simulink library "ox_lib"  (Simulink 7.5)
settings: Solver=ode45  SolverMode=SingleTasking  StartTime=0.0  StopTime=10.0  RelTol=1e-3
PostLoadFcn:
  | % Stub definitions for mask variables
  | delay_depth=16;
  | n_bits=8;
  | bin_pt=7;
libraries: xbsIndex_r4 x493, casper_library x127, casper_library_misc x2, xps_library x2, casper_library_delays x1
(part 3 of 5)

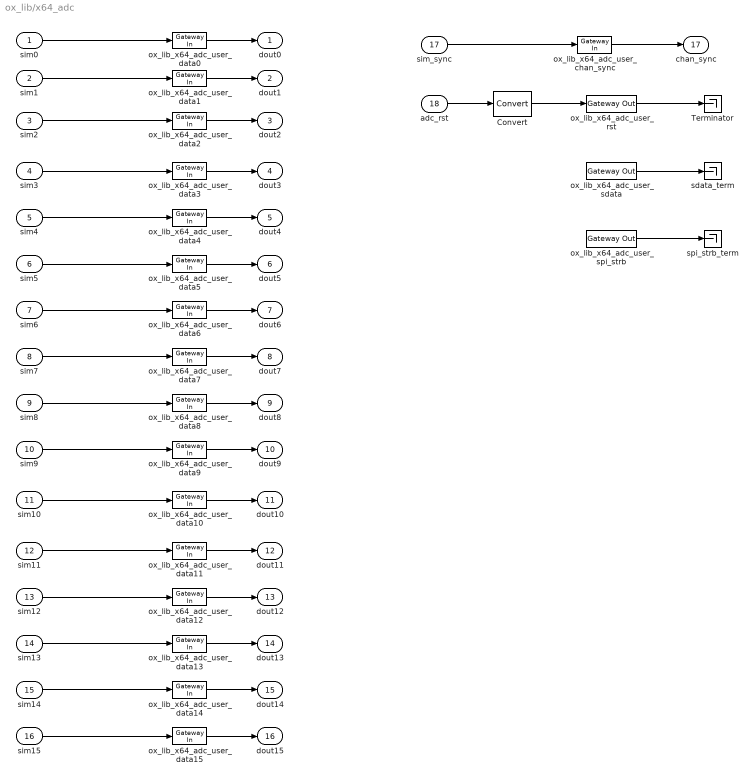
== system ox_lib/x64_adc ==
  sim0 : Inport
  sim1 : Inport  Port=2
  sim2 : Inport  Port=3
  sim3 : Inport  Port=4
  sim4 : Inport  Port=5
  sim5 : Inport  Port=6
  sim6 : Inport  Port=7
  sim7 : Inport  Port=8
  sim8 : Inport  Port=9
  sim9 : Inport  Port=10
  sim10 : Inport  Port=11
  sim11 : Inport  Port=12
  sim12 : Inport  Port=13
  sim13 : Inport  Port=14
  sim14 : Inport  Port=15
  sim15 : Inport  Port=16
  sim_sync : Inport  Port=17
  adc_rst : Inport  Port=18
  Convert : xbsIndex_r4/Convert  arith_type=Boolean  n_bits=16  bin_pt=14  quantization=Truncate  overflow=Wrap  latency=0  dbl_ovrd=off  pipeline=off  block_type=convert
      settings: block_version=11.4
  Terminator : Terminator
  ox_lib_x64_adc_user_chan_sync : xbsIndex_r4/Gateway In  arith_type=Unsigned  n_bits=8  bin_pt=0  quantization="Round  (unbiased: +/- Inf)"  overflow=Saturate  period=1  dbl_ovrd=off  timing_constraint=None  locs_specified=off  LOCs={}  hdl_port=on  block_type=gatewayin
      settings: infoedit="Gateway in block.  Converts inputs of type Simulink integer, double and fixed point to  Xilinx fixed point type.<br><br>Hardware notes:  In hardware these blocks become top level input ports."  block_version=11.4
  ox_lib_x64_adc_user_data{0..15} (16 alike) : xbsIndex_r4/Gateway In  arith_type="Signed  (2's comp)"  n_bits=12  bin_pt=11  quantization="Round  (unbiased: +/- Inf)"  overflow=Saturate  period=1  dbl_ovrd=off  timing_constraint=None  locs_specified=off  LOCs={}  hdl_port=on  block_type=gatewayin
      settings: infoedit="Gateway in block.  Converts inputs of type Simulink integer, double and fixed point to  Xilinx fixed point type.<br><br>Hardware notes:  In hardware these blocks become top level input ports."  block_version=11.4
  ox_lib_x64_adc_user_rst : xbsIndex_r4/Gateway Out  hdl_port=on  timing_constraint=None  locs_specified=off  LOCs={}  block_type=gatewayout
      settings: infoedit="Gateway out block.  Converts Xilinx fixed point inputs into ouputs of type Simulink integer, double, or fixed point.<br><br>Hardware notes:  In hardware these blocks become top level output ports or are discarded, depending on how they are configured."  block_version=11.4
  ox_lib_x64_adc_user_sdata : xbsIndex_r4/Gateway Out  hdl_port=on  timing_constraint=None  locs_specified=off  LOCs={}  block_type=gatewayout
      settings: infoedit="Gateway out block.  Converts Xilinx fixed point inputs into ouputs of type Simulink integer, double, or fixed point.<br><br>Hardware notes:  In hardware these blocks become top level output ports or are discarded, depending on how they are configured."  block_version=11.4
  ox_lib_x64_adc_user_spi_strb : xbsIndex_r4/Gateway Out  hdl_port=on  timing_constraint=None  locs_specified=off  LOCs={}  block_type=gatewayout
      settings: infoedit="Gateway out block.  Converts Xilinx fixed point inputs into ouputs of type Simulink integer, double, or fixed point.<br><br>Hardware notes:  In hardware these blocks become top level output ports or are discarded, depending on how they are configured."  block_version=11.4
  sdata_term : Terminator
  spi_strb_term : Terminator
  dout0 : Outport
  dout1 : Outport  Port=2
  dout2 : Outport  Port=3
  dout3 : Outport  Port=4
  dout4 : Outport  Port=5
  dout5 : Outport  Port=6
  dout6 : Outport  Port=7
  dout7 : Outport  Port=8
  dout8 : Outport  Port=9
  dout9 : Outport  Port=10
  dout10 : Outport  Port=11
  dout11 : Outport  Port=12
  dout12 : Outport  Port=13
  dout13 : Outport  Port=14
  dout14 : Outport  Port=15
  dout15 : Outport  Port=16
  chan_sync : Outport  Port=17
  wires:
  ox_lib_x64_adc_user_data1/1 -> dout1/1
  sim1/1 -> ox_lib_x64_adc_user_data1/1
  Convert/1 -> ox_lib_x64_adc_user_rst/1
  ox_lib_x64_adc_user_rst/1 -> Terminator/1
  adc_rst/1 -> Convert/1
  ox_lib_x64_adc_user_chan_sync/1 -> chan_sync/1
  sim_sync/1 -> ox_lib_x64_adc_user_chan_sync/1
  ox_lib_x64_adc_user_data15/1 -> dout15/1
  sim15/1 -> ox_lib_x64_adc_user_data15/1
  ox_lib_x64_adc_user_data14/1 -> dout14/1
  sim14/1 -> ox_lib_x64_adc_user_data14/1
  ox_lib_x64_adc_user_data13/1 -> dout13/1
  sim13/1 -> ox_lib_x64_adc_user_data13/1
  ox_lib_x64_adc_user_data12/1 -> dout12/1
  sim12/1 -> ox_lib_x64_adc_user_data12/1
  ox_lib_x64_adc_user_data11/1 -> dout11/1
  sim11/1 -> ox_lib_x64_adc_user_data11/1
  ox_lib_x64_adc_user_data10/1 -> dout10/1
  sim10/1 -> ox_lib_x64_adc_user_data10/1
  ox_lib_x64_adc_user_data9/1 -> dout9/1
  sim9/1 -> ox_lib_x64_adc_user_data9/1
  ox_lib_x64_adc_user_data8/1 -> dout8/1
  sim8/1 -> ox_lib_x64_adc_user_data8/1
  ox_lib_x64_adc_user_data7/1 -> dout7/1
  sim7/1 -> ox_lib_x64_adc_user_data7/1
  ox_lib_x64_adc_user_data6/1 -> dout6/1
  sim6/1 -> ox_lib_x64_adc_user_data6/1
  ox_lib_x64_adc_user_data5/1 -> dout5/1
  sim5/1 -> ox_lib_x64_adc_user_data5/1
  ox_lib_x64_adc_user_data4/1 -> dout4/1
  sim4/1 -> ox_lib_x64_adc_user_data4/1
  ox_lib_x64_adc_user_data3/1 -> dout3/1
  sim3/1 -> ox_lib_x64_adc_user_data3/1
  ox_lib_x64_adc_user_data2/1 -> dout2/1
  sim2/1 -> ox_lib_x64_adc_user_data2/1
  ox_lib_x64_adc_user_data0/1 -> dout0/1
  sim0/1 -> ox_lib_x64_adc_user_data0/1
  ? -> ox_lib_x64_adc_user_sdata/1
  ? -> ox_lib_x64_adc_user_spi_strb/1
  ox_lib_x64_adc_user_sdata/1 -> sdata_term/1
  ox_lib_x64_adc_user_spi_strb/1 -> spi_strb_term/1

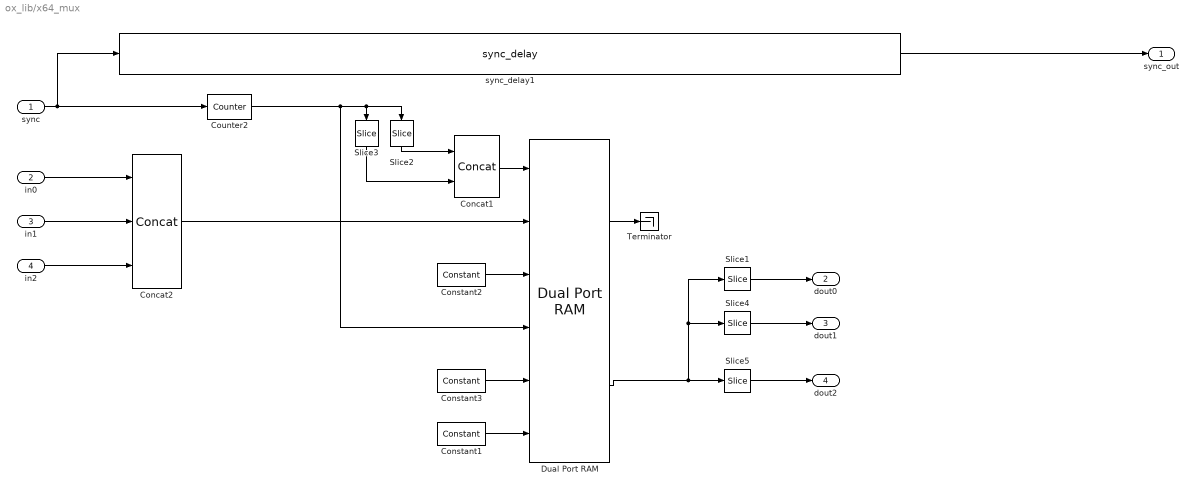
== system ox_lib/x64_mux ==
  sync : Inport  OutDataType=fixdt(1, 16)  OutScaling=2^0
  in0 : Inport  Port=2  OutDataType=fixdt(1, 16)  OutScaling=2^0
  in1 : Inport  Port=3  OutDataType=fixdt(1, 16)  OutScaling=2^0
  in2 : Inport  Port=4  OutDataType=fixdt(1, 16)  OutScaling=2^0
  Concat1 : xbsIndex_r4/Concat  num_inputs=2  dbl_ovrd=off  block_type=concat
  Concat2 : xbsIndex_r4/Concat  num_inputs=3  dbl_ovrd=off  block_type=concat
  Constant1 : xbsIndex_r4/Constant  arith_type=Boolean  const=0  n_bits=16  bin_pt=14  explicit_period=off  period=1  equ=P=C  opselect=C  inp2=PCIN>>17  opr=+  inp1=P  carry=CIN  dbl_ovrd=off  block_type=constant
      settings: block_version=11.4
  Constant2 : xbsIndex_r4/Constant  arith_type=Boolean  const=1  n_bits=16  bin_pt=14  explicit_period=on  period=1  equ=P=C  opselect=C  inp2=PCIN>>17  opr=+  inp1=P  carry=CIN  dbl_ovrd=off  block_type=constant
      settings: block_version=11.4
  Constant3 : xbsIndex_r4/Constant  arith_type=Unsigned  const=0  n_bits=36  bin_pt=0  explicit_period=on  period=1  equ=P=C  opselect=C  inp2=PCIN>>17  opr=+  inp1=P  carry=CIN  dbl_ovrd=off  block_type=constant
      settings: block_version=11.4
  Counter2 : xbsIndex_r4/Counter  cnt_type=Free Running  cnt_to=Inf  operation=Up  start_count=0  cnt_by_val=1  arith_type=Unsigned  n_bits=fft_len+2  bin_pt=0  load_pin=off  rst=on  en=off  explicit_period=on  period=1  dbl_ovrd=off  use_behavioral_HDL=off  implementation=Fabric  block_type=counter
      settings: block_version=11.4
  Dual Port RAM : xbsIndex_r4/Dual Port RAM  depth=2^(fft_len+2)  initVector=0  distributed_mem=Block RAM  init_a=0  init_b=0  rst_a=off  rst_b=off  en_a=off  en_b=off  latency=bram_lat  write_mode_A=Read Before Write  write_mode_B=Read Before Write  dbl_ovrd=off  optimize=Area  use_rpm=on  block_type=dpram
      settings: block_version=11.4
  Slice1 : xbsIndex_r4/Slice  nbits=12  boolean_output=off  mode=Lower Bit Location + Width  bit1=0  base1=MSB of Input  bit0=24  base0=LSB of Input  dbl_ovrd=off  block_type=slice
  Slice2 : xbsIndex_r4/Slice  nbits=2  boolean_output=off  mode=Lower Bit Location + Width  bit1=0  base1=MSB of Input  bit0=0  base0=LSB of Input  dbl_ovrd=off  block_type=slice
  Slice3 : xbsIndex_r4/Slice  nbits=fft_len  boolean_output=off  mode=Lower Bit Location + Width  bit1=0  base1=MSB of Input  bit0=2  base0=LSB of Input  dbl_ovrd=off  block_type=slice
  Slice4 : xbsIndex_r4/Slice  nbits=12  boolean_output=off  mode=Lower Bit Location + Width  bit1=0  base1=MSB of Input  bit0=12  base0=LSB of Input  dbl_ovrd=off  block_type=slice
  Slice5 : xbsIndex_r4/Slice  nbits=12  boolean_output=off  mode=Lower Bit Location + Width  bit1=0  base1=MSB of Input  bit0=0  base0=LSB of Input  dbl_ovrd=off  block_type=slice
  Terminator : Terminator
  sync_delay1 : casper_library/Delays/sync_delay  SystemSampleTime=-1  DelayLen=2^(fft_len+2)+bram_lat
  sync_out : Outport
  dout0 : Outport  Port=2
  dout1 : Outport  Port=3
  dout2 : Outport  Port=4
  wires:
  sync/1 -> Counter2/1, sync_delay1/1
  Counter2/1 -> Slice2/1, Slice3/1, Dual Port RAM/4
  Constant1/1 -> Dual Port RAM/6
  Constant3/1 -> Dual Port RAM/5
  sync_delay1/1 -> sync_out/1
  Dual Port RAM/1 -> Terminator/1
  in0/1 -> Concat2/1
  in1/1 -> Concat2/2
  in2/1 -> Concat2/3
  Slice2/1 -> Concat1/1
  Slice3/1 -> Concat1/2
  Concat1/1 -> Dual Port RAM/1
  Dual Port RAM/2 -> Slice5/1, Slice4/1, Slice1/1
  Slice5/1 -> dout2/1
  Slice1/1 -> dout0/1
  Slice4/1 -> dout1/1
  Concat2/1 -> Dual Port RAM/2
  Constant2/1 -> Dual Port RAM/3

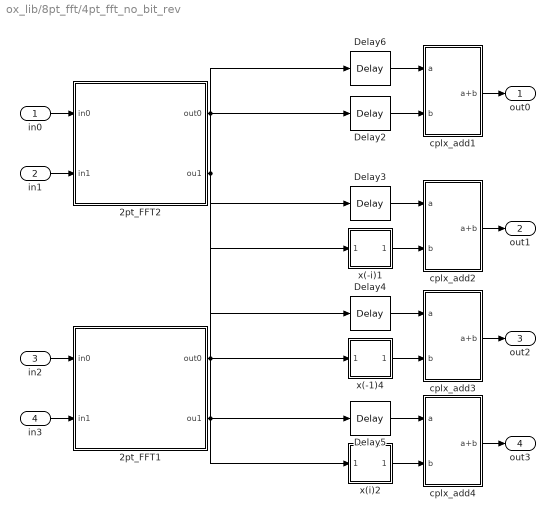
== system ox_lib/8pt_fft/4pt_fft_no_bit_rev ==
  in0 : Inport
  in1 : Inport  Port=2
  in2 : Inport  Port=3
  in3 : Inport  Port=4
  2pt_FFT1 : Subsystem
  2pt_FFT2 : Subsystem
  Delay{2..6} (5 alike) : xbsIndex_r4/Delay  en=off  latency=2  dbl_ovrd=off  reg_retiming=off  block_type=delay
      settings: block_version=11.4
  cplx_add1 : Subsystem  AncestorBlock=casper_library/Misc/complex_addsub  mask(cplx_add){BitWidth=8, add_latency=2}
      mask prompts: BitWidth "Bit Wdith"; add_latency "Add Latency"
  cplx_add2 : Subsystem  AncestorBlock=casper_library/Misc/complex_addsub  mask(cplx_add){BitWidth=8, add_latency=2}
      mask prompts: BitWidth "Bit Wdith"; add_latency "Add Latency"
  cplx_add3 : Subsystem  AncestorBlock=casper_library/Misc/complex_addsub  mask(cplx_add){BitWidth=8, add_latency=2}
      mask prompts: BitWidth "Bit Wdith"; add_latency "Add Latency"
  cplx_add4 : Subsystem  AncestorBlock=casper_library/Misc/complex_addsub  mask(cplx_add){BitWidth=8, add_latency=2}
      mask prompts: BitWidth "Bit Wdith"; add_latency "Add Latency"
  x(-1)4 : Subsystem
  x(-i)1 : Subsystem
  x(i)2 : Subsystem
  out0 : Outport
  out1 : Outport  Port=2
  out2 : Outport  Port=3
  out3 : Outport  Port=4
  wires:
  cplx_add4/1(a+b) -> out3/1
  in3/1 -> 2pt_FFT1/2(in1)
  in2/1 -> 2pt_FFT1/1(in0)
  cplx_add3/1(a+b) -> out2/1
  cplx_add2/1(a+b) -> out1/1
  in1/1 -> 2pt_FFT2/2(in1)
  in0/1 -> 2pt_FFT2/1(in0)
  cplx_add1/1(a+b) -> out0/1
  x(i)2/1(Out1) -> cplx_add4/2(b)
  Delay5/1 -> cplx_add4/1(a)
  x(-1)4/1(Out1) -> cplx_add3/2(b)
  Delay4/1 -> cplx_add3/1(a)
  x(-i)1/1(Out1) -> cplx_add2/2(b)
  Delay3/1 -> cplx_add2/1(a)
  Delay2/1 -> cplx_add1/2(b)
  Delay6/1 -> cplx_add1/1(a)
  2pt_FFT2/1(out0) -> Delay6/1, Delay4/1
  2pt_FFT2/2(ou1) -> Delay5/1, Delay3/1
  2pt_FFT1/1(out0) -> x(-1)4/1(In1), Delay2/1
  2pt_FFT1/2(ou1) -> x(-i)1/1(In1), x(i)2/1(In1)

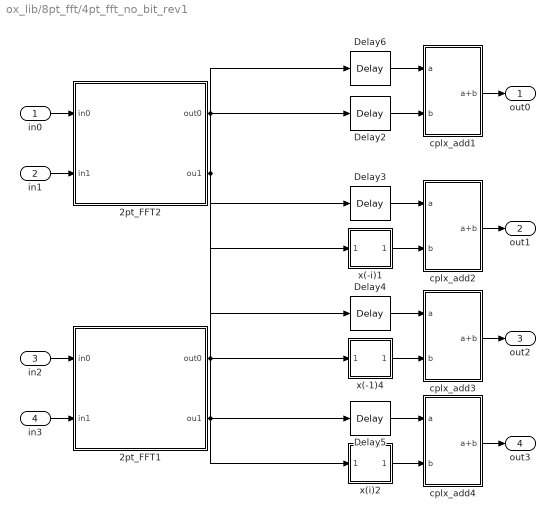
== system ox_lib/8pt_fft/4pt_fft_no_bit_rev1 ==
  in0 : Inport
  in1 : Inport  Port=2
  in2 : Inport  Port=3
  in3 : Inport  Port=4
  2pt_FFT1 : Subsystem
  2pt_FFT2 : Subsystem
  Delay{2..6} (5 alike) : xbsIndex_r4/Delay  en=off  latency=2  dbl_ovrd=off  reg_retiming=off  block_type=delay
      settings: block_version=11.4
  cplx_add1 : Subsystem  AncestorBlock=casper_library/Misc/complex_addsub  mask(cplx_add){BitWidth=8, add_latency=2}
      mask prompts: BitWidth "Bit Wdith"; add_latency "Add Latency"
  cplx_add2 : Subsystem  AncestorBlock=casper_library/Misc/complex_addsub  mask(cplx_add){BitWidth=8, add_latency=2}
      mask prompts: BitWidth "Bit Wdith"; add_latency "Add Latency"
  cplx_add3 : Subsystem  AncestorBlock=casper_library/Misc/complex_addsub  mask(cplx_add){BitWidth=8, add_latency=2}
      mask prompts: BitWidth "Bit Wdith"; add_latency "Add Latency"
  cplx_add4 : Subsystem  AncestorBlock=casper_library/Misc/complex_addsub  mask(cplx_add){BitWidth=8, add_latency=2}
      mask prompts: BitWidth "Bit Wdith"; add_latency "Add Latency"
  x(-1)4 : Subsystem
  x(-i)1 : Subsystem
  x(i)2 : Subsystem
  out0 : Outport
  out1 : Outport  Port=2
  out2 : Outport  Port=3
  out3 : Outport  Port=4
  wires:
  2pt_FFT1/2(ou1) -> x(i)2/1(In1), x(-i)1/1(In1)
  2pt_FFT1/1(out0) -> Delay2/1, x(-1)4/1(In1)
  2pt_FFT2/2(ou1) -> Delay3/1, Delay5/1
  2pt_FFT2/1(out0) -> Delay4/1, Delay6/1
  Delay6/1 -> cplx_add1/1(a)
  Delay2/1 -> cplx_add1/2(b)
  Delay3/1 -> cplx_add2/1(a)
  x(-i)1/1(Out1) -> cplx_add2/2(b)
  Delay4/1 -> cplx_add3/1(a)
  x(-1)4/1(Out1) -> cplx_add3/2(b)
  Delay5/1 -> cplx_add4/1(a)
  x(i)2/1(Out1) -> cplx_add4/2(b)
  cplx_add1/1(a+b) -> out0/1
  in0/1 -> 2pt_FFT2/1(in0)
  in1/1 -> 2pt_FFT2/2(in1)
  cplx_add2/1(a+b) -> out1/1
  cplx_add3/1(a+b) -> out2/1
  in2/1 -> 2pt_FFT1/1(in0)
  in3/1 -> 2pt_FFT1/2(in1)
  cplx_add4/1(a+b) -> out3/1

== system ox_lib/8pt_fft/cplx_add1 ==
  a : Inport  OutDataType=sfix(16)  OutScaling=2^0
  b : Inport  Port=2  OutDataType=sfix(16)  OutScaling=2^0
  AddSub : xbsIndex_r4/AddSub  mode=Addition  use_carryin=off  use_carryout=off  en=off  latency=add_latency  precision=Full  arith_type=Unsigned  n_bits=8  bin_pt=2  quantization=Truncate  overflow=Wrap  dbl_ovrd=off  use_behavioral_HDL=on  hw_selection=Fabric  pipelined=off  use_rpm=on  block_type=addsub
      settings: xl_area=[0, 0, 0, 0, 0, 0, 0]  block_version=9.1.01
  AddSub2 : xbsIndex_r4/AddSub  mode=Addition  use_carryin=off  use_carryout=off  en=off  latency=add_latency  precision=Full  arith_type=Unsigned  n_bits=8  bin_pt=2  quantization=Truncate  overflow=Wrap  dbl_ovrd=off  use_behavioral_HDL=on  hw_selection=Fabric  pipelined=off  use_rpm=on  block_type=addsub
      settings: xl_area=[0, 0, 0, 0, 0, 0, 0]  block_version=9.1.01
  Convert : xbsIndex_r4/Convert  arith_type="Signed  (2's comp)"  n_bits=BitWidth  bin_pt=BitWidth - 1  quantization="Round  (unbiased: +/- Inf)"  overflow=Saturate  latency=add_latency  dbl_ovrd=off  pipeline=off  block_type=convert
      settings: xl_area=[0, 0, 0, 0, 0, 0, 0]
  Convert2 : xbsIndex_r4/Convert  arith_type="Signed  (2's comp)"  n_bits=BitWidth  bin_pt=BitWidth - 1  quantization="Round  (unbiased: +/- Inf)"  overflow=Saturate  latency=add_latency  dbl_ovrd=off  pipeline=off  block_type=convert
      settings: xl_area=[0, 0, 0, 0, 0, 0, 0]
  Scale : xbsIndex_r4/Scale  scale_factor=-1  dbl_ovrd=off  block_type=scale
  Scale1 : xbsIndex_r4/Scale  scale_factor=-1  dbl_ovrd=off  block_type=scale
  c_to_ri : casper_library/Misc/c_to_ri  SystemSampleTime=-1  n_bits=BitWidth  bin_pt=BitWidth-1
      settings: AttributesFormatString=8_7 r/i
  c_to_ri1 : casper_library/Misc/c_to_ri  SystemSampleTime=-1  n_bits=BitWidth  bin_pt=BitWidth-1
      settings: AttributesFormatString=8_7 r/i
  ri_to_c : casper_library/Misc/ri_to_c  SystemSampleTime=-1
  a+b : Outport  OutDataType=sfix(16)  OutScaling=2^0
  wires:
  AddSub/1 -> Scale1/1
  AddSub2/1 -> Scale/1
  c_to_ri/1 -> AddSub/1
  c_to_ri/2 -> AddSub2/1
  c_to_ri1/1 -> AddSub/2
  c_to_ri1/2 -> AddSub2/2
  Convert/1 -> ri_to_c/1
  Convert2/1 -> ri_to_c/2
  a/1 -> c_to_ri/1
  ri_to_c/1 -> a+b/1
  b/1 -> c_to_ri1/1
  Scale1/1 -> Convert/1
  Scale/1 -> Convert2/1

== system ox_lib/8pt_fft/cplx_add2 ==
  a : Inport  OutDataType=sfix(16)  OutScaling=2^0
  b : Inport  Port=2  OutDataType=sfix(16)  OutScaling=2^0
  AddSub : xbsIndex_r4/AddSub  mode=Addition  use_carryin=off  use_carryout=off  en=off  latency=add_latency  precision=Full  arith_type=Unsigned  n_bits=8  bin_pt=2  quantization=Truncate  overflow=Wrap  dbl_ovrd=off  use_behavioral_HDL=on  hw_selection=Fabric  pipelined=off  use_rpm=on  block_type=addsub
      settings: xl_area=[0, 0, 0, 0, 0, 0, 0]  block_version=9.1.01
  AddSub2 : xbsIndex_r4/AddSub  mode=Addition  use_carryin=off  use_carryout=off  en=off  latency=add_latency  precision=Full  arith_type=Unsigned  n_bits=8  bin_pt=2  quantization=Truncate  overflow=Wrap  dbl_ovrd=off  use_behavioral_HDL=on  hw_selection=Fabric  pipelined=off  use_rpm=on  block_type=addsub
      settings: xl_area=[0, 0, 0, 0, 0, 0, 0]  block_version=9.1.01
  Convert : xbsIndex_r4/Convert  arith_type="Signed  (2's comp)"  n_bits=BitWidth  bin_pt=BitWidth - 1  quantization="Round  (unbiased: +/- Inf)"  overflow=Saturate  latency=add_latency  dbl_ovrd=off  pipeline=off  block_type=convert
      settings: xl_area=[0, 0, 0, 0, 0, 0, 0]
  Convert2 : xbsIndex_r4/Convert  arith_type="Signed  (2's comp)"  n_bits=BitWidth  bin_pt=BitWidth - 1  quantization="Round  (unbiased: +/- Inf)"  overflow=Saturate  latency=add_latency  dbl_ovrd=off  pipeline=off  block_type=convert
      settings: xl_area=[0, 0, 0, 0, 0, 0, 0]
  Scale : xbsIndex_r4/Scale  scale_factor=-1  dbl_ovrd=off  block_type=scale
  Scale1 : xbsIndex_r4/Scale  scale_factor=-1  dbl_ovrd=off  block_type=scale
  c_to_ri : casper_library/Misc/c_to_ri  SystemSampleTime=-1  n_bits=BitWidth  bin_pt=BitWidth-1
      settings: AttributesFormatString=8_7 r/i
  c_to_ri1 : casper_library/Misc/c_to_ri  SystemSampleTime=-1  n_bits=BitWidth  bin_pt=BitWidth-1
      settings: AttributesFormatString=8_7 r/i
  ri_to_c : casper_library/Misc/ri_to_c  SystemSampleTime=-1
  a+b : Outport  OutDataType=sfix(16)  OutScaling=2^0
  wires:
  Scale/1 -> Convert2/1
  Scale1/1 -> Convert/1
  b/1 -> c_to_ri1/1
  ri_to_c/1 -> a+b/1
  a/1 -> c_to_ri/1
  Convert2/1 -> ri_to_c/2
  Convert/1 -> ri_to_c/1
  c_to_ri1/2 -> AddSub2/2
  c_to_ri1/1 -> AddSub/2
  c_to_ri/2 -> AddSub2/1
  c_to_ri/1 -> AddSub/1
  AddSub2/1 -> Scale/1
  AddSub/1 -> Scale1/1

== system ox_lib/8pt_fft/cplx_add3 ==
  a : Inport  OutDataType=sfix(16)  OutScaling=2^0
  b : Inport  Port=2  OutDataType=sfix(16)  OutScaling=2^0
  AddSub : xbsIndex_r4/AddSub  mode=Addition  use_carryin=off  use_carryout=off  en=off  latency=add_latency  precision=Full  arith_type=Unsigned  n_bits=8  bin_pt=2  quantization=Truncate  overflow=Wrap  dbl_ovrd=off  use_behavioral_HDL=on  hw_selection=Fabric  pipelined=off  use_rpm=on  block_type=addsub
      settings: xl_area=[0, 0, 0, 0, 0, 0, 0]  block_version=9.1.01
  AddSub2 : xbsIndex_r4/AddSub  mode=Addition  use_carryin=off  use_carryout=off  en=off  latency=add_latency  precision=Full  arith_type=Unsigned  n_bits=8  bin_pt=2  quantization=Truncate  overflow=Wrap  dbl_ovrd=off  use_behavioral_HDL=on  hw_selection=Fabric  pipelined=off  use_rpm=on  block_type=addsub
      settings: xl_area=[0, 0, 0, 0, 0, 0, 0]  block_version=9.1.01
  Convert : xbsIndex_r4/Convert  arith_type="Signed  (2's comp)"  n_bits=BitWidth  bin_pt=BitWidth - 1  quantization="Round  (unbiased: +/- Inf)"  overflow=Saturate  latency=add_latency  dbl_ovrd=off  pipeline=off  block_type=convert
      settings: xl_area=[0, 0, 0, 0, 0, 0, 0]
  Convert2 : xbsIndex_r4/Convert  arith_type="Signed  (2's comp)"  n_bits=BitWidth  bin_pt=BitWidth - 1  quantization="Round  (unbiased: +/- Inf)"  overflow=Saturate  latency=add_latency  dbl_ovrd=off  pipeline=off  block_type=convert
      settings: xl_area=[0, 0, 0, 0, 0, 0, 0]
  Scale : xbsIndex_r4/Scale  scale_factor=-1  dbl_ovrd=off  block_type=scale
  Scale1 : xbsIndex_r4/Scale  scale_factor=-1  dbl_ovrd=off  block_type=scale
  c_to_ri : casper_library/Misc/c_to_ri  SystemSampleTime=-1  n_bits=BitWidth  bin_pt=BitWidth-1
      settings: AttributesFormatString=8_7 r/i
  c_to_ri1 : casper_library/Misc/c_to_ri  SystemSampleTime=-1  n_bits=BitWidth  bin_pt=BitWidth-1
      settings: AttributesFormatString=8_7 r/i
  ri_to_c : casper_library/Misc/ri_to_c  SystemSampleTime=-1
  a+b : Outport  OutDataType=sfix(16)  OutScaling=2^0
  wires:
  AddSub/1 -> Scale1/1
  AddSub2/1 -> Scale/1
  c_to_ri/1 -> AddSub/1
  c_to_ri/2 -> AddSub2/1
  c_to_ri1/1 -> AddSub/2
  c_to_ri1/2 -> AddSub2/2
  Convert/1 -> ri_to_c/1
  Convert2/1 -> ri_to_c/2
  a/1 -> c_to_ri/1
  ri_to_c/1 -> a+b/1
  b/1 -> c_to_ri1/1
  Scale1/1 -> Convert/1
  Scale/1 -> Convert2/1

== system ox_lib/8pt_fft/cplx_add4 ==
  a : Inport  OutDataType=sfix(16)  OutScaling=2^0
  b : Inport  Port=2  OutDataType=sfix(16)  OutScaling=2^0
  AddSub : xbsIndex_r4/AddSub  mode=Addition  use_carryin=off  use_carryout=off  en=off  latency=add_latency  precision=Full  arith_type=Unsigned  n_bits=8  bin_pt=2  quantization=Truncate  overflow=Wrap  dbl_ovrd=off  use_behavioral_HDL=on  hw_selection=Fabric  pipelined=off  use_rpm=on  block_type=addsub
      settings: xl_area=[0, 0, 0, 0, 0, 0, 0]  block_version=9.1.01
  AddSub2 : xbsIndex_r4/AddSub  mode=Addition  use_carryin=off  use_carryout=off  en=off  latency=add_latency  precision=Full  arith_type=Unsigned  n_bits=8  bin_pt=2  quantization=Truncate  overflow=Wrap  dbl_ovrd=off  use_behavioral_HDL=on  hw_selection=Fabric  pipelined=off  use_rpm=on  block_type=addsub
      settings: xl_area=[0, 0, 0, 0, 0, 0, 0]  block_version=9.1.01
  Convert : xbsIndex_r4/Convert  arith_type="Signed  (2's comp)"  n_bits=BitWidth  bin_pt=BitWidth - 1  quantization="Round  (unbiased: +/- Inf)"  overflow=Saturate  latency=add_latency  dbl_ovrd=off  pipeline=off  block_type=convert
      settings: xl_area=[0, 0, 0, 0, 0, 0, 0]
  Convert2 : xbsIndex_r4/Convert  arith_type="Signed  (2's comp)"  n_bits=BitWidth  bin_pt=BitWidth - 1  quantization="Round  (unbiased: +/- Inf)"  overflow=Saturate  latency=add_latency  dbl_ovrd=off  pipeline=off  block_type=convert
      settings: xl_area=[0, 0, 0, 0, 0, 0, 0]
  Scale : xbsIndex_r4/Scale  scale_factor=-1  dbl_ovrd=off  block_type=scale
  Scale1 : xbsIndex_r4/Scale  scale_factor=-1  dbl_ovrd=off  block_type=scale
  c_to_ri : casper_library/Misc/c_to_ri  SystemSampleTime=-1  n_bits=BitWidth  bin_pt=BitWidth-1
      settings: AttributesFormatString=8_7 r/i
  c_to_ri1 : casper_library/Misc/c_to_ri  SystemSampleTime=-1  n_bits=BitWidth  bin_pt=BitWidth-1
      settings: AttributesFormatString=8_7 r/i
  ri_to_c : casper_library/Misc/ri_to_c  SystemSampleTime=-1
  a+b : Outport  OutDataType=sfix(16)  OutScaling=2^0
  wires:
  Scale/1 -> Convert2/1
  Scale1/1 -> Convert/1
  b/1 -> c_to_ri1/1
  ri_to_c/1 -> a+b/1
  a/1 -> c_to_ri/1
  Convert2/1 -> ri_to_c/2
  Convert/1 -> ri_to_c/1
  c_to_ri1/2 -> AddSub2/2
  c_to_ri1/1 -> AddSub/2
  c_to_ri/2 -> AddSub2/1
  c_to_ri/1 -> AddSub/1
  AddSub2/1 -> Scale/1
  AddSub/1 -> Scale1/1

== system ox_lib/8pt_fft/cplx_add5 ==
  a : Inport  OutDataType=sfix(16)  OutScaling=2^0
  b : Inport  Port=2  OutDataType=sfix(16)  OutScaling=2^0
  AddSub : xbsIndex_r4/AddSub  mode=Addition  use_carryin=off  use_carryout=off  en=off  latency=add_latency  precision=Full  arith_type=Unsigned  n_bits=8  bin_pt=2  quantization=Truncate  overflow=Wrap  dbl_ovrd=off  use_behavioral_HDL=on  hw_selection=Fabric  pipelined=off  use_rpm=on  block_type=addsub
      settings: xl_area=[0, 0, 0, 0, 0, 0, 0]  block_version=9.1.01
  AddSub2 : xbsIndex_r4/AddSub  mode=Addition  use_carryin=off  use_carryout=off  en=off  latency=add_latency  precision=Full  arith_type=Unsigned  n_bits=8  bin_pt=2  quantization=Truncate  overflow=Wrap  dbl_ovrd=off  use_behavioral_HDL=on  hw_selection=Fabric  pipelined=off  use_rpm=on  block_type=addsub
      settings: xl_area=[0, 0, 0, 0, 0, 0, 0]  block_version=9.1.01
  Convert : xbsIndex_r4/Convert  arith_type="Signed  (2's comp)"  n_bits=BitWidth  bin_pt=BitWidth - 1  quantization="Round  (unbiased: +/- Inf)"  overflow=Saturate  latency=add_latency  dbl_ovrd=off  pipeline=off  block_type=convert
      settings: xl_area=[0, 0, 0, 0, 0, 0, 0]
  Convert2 : xbsIndex_r4/Convert  arith_type="Signed  (2's comp)"  n_bits=BitWidth  bin_pt=BitWidth - 1  quantization="Round  (unbiased: +/- Inf)"  overflow=Saturate  latency=add_latency  dbl_ovrd=off  pipeline=off  block_type=convert
      settings: xl_area=[0, 0, 0, 0, 0, 0, 0]
  Scale : xbsIndex_r4/Scale  scale_factor=-1  dbl_ovrd=off  block_type=scale
  Scale1 : xbsIndex_r4/Scale  scale_factor=-1  dbl_ovrd=off  block_type=scale
  c_to_ri : casper_library/Misc/c_to_ri  SystemSampleTime=-1  n_bits=BitWidth  bin_pt=BitWidth-1
      settings: AttributesFormatString=8_7 r/i
  c_to_ri1 : casper_library/Misc/c_to_ri  SystemSampleTime=-1  n_bits=BitWidth  bin_pt=BitWidth-1
      settings: AttributesFormatString=8_7 r/i
  ri_to_c : casper_library/Misc/ri_to_c  SystemSampleTime=-1
  a+b : Outport  OutDataType=sfix(16)  OutScaling=2^0
  wires:
  AddSub/1 -> Scale1/1
  AddSub2/1 -> Scale/1
  c_to_ri/1 -> AddSub/1
  c_to_ri/2 -> AddSub2/1
  c_to_ri1/1 -> AddSub/2
  c_to_ri1/2 -> AddSub2/2
  Convert/1 -> ri_to_c/1
  Convert2/1 -> ri_to_c/2
  a/1 -> c_to_ri/1
  ri_to_c/1 -> a+b/1
  b/1 -> c_to_ri1/1
  Scale1/1 -> Convert/1
  Scale/1 -> Convert2/1

== system ox_lib/8pt_fft/cplx_add6 ==
  a : Inport  OutDataType=sfix(16)  OutScaling=2^0
  b : Inport  Port=2  OutDataType=sfix(16)  OutScaling=2^0
  AddSub : xbsIndex_r4/AddSub  mode=Addition  use_carryin=off  use_carryout=off  en=off  latency=add_latency  precision=Full  arith_type=Unsigned  n_bits=8  bin_pt=2  quantization=Truncate  overflow=Wrap  dbl_ovrd=off  use_behavioral_HDL=on  hw_selection=Fabric  pipelined=off  use_rpm=on  block_type=addsub
      settings: xl_area=[0, 0, 0, 0, 0, 0, 0]  block_version=9.1.01
  AddSub2 : xbsIndex_r4/AddSub  mode=Addition  use_carryin=off  use_carryout=off  en=off  latency=add_latency  precision=Full  arith_type=Unsigned  n_bits=8  bin_pt=2  quantization=Truncate  overflow=Wrap  dbl_ovrd=off  use_behavioral_HDL=on  hw_selection=Fabric  pipelined=off  use_rpm=on  block_type=addsub
      settings: xl_area=[0, 0, 0, 0, 0, 0, 0]  block_version=9.1.01
  Convert : xbsIndex_r4/Convert  arith_type="Signed  (2's comp)"  n_bits=BitWidth  bin_pt=BitWidth - 1  quantization="Round  (unbiased: +/- Inf)"  overflow=Saturate  latency=add_latency  dbl_ovrd=off  pipeline=off  block_type=convert
      settings: xl_area=[0, 0, 0, 0, 0, 0, 0]
  Convert2 : xbsIndex_r4/Convert  arith_type="Signed  (2's comp)"  n_bits=BitWidth  bin_pt=BitWidth - 1  quantization="Round  (unbiased: +/- Inf)"  overflow=Saturate  latency=add_latency  dbl_ovrd=off  pipeline=off  block_type=convert
      settings: xl_area=[0, 0, 0, 0, 0, 0, 0]
  Scale : xbsIndex_r4/Scale  scale_factor=-1  dbl_ovrd=off  block_type=scale
  Scale1 : xbsIndex_r4/Scale  scale_factor=-1  dbl_ovrd=off  block_type=scale
  c_to_ri : casper_library/Misc/c_to_ri  SystemSampleTime=-1  n_bits=BitWidth  bin_pt=BitWidth-1
      settings: AttributesFormatString=8_7 r/i
  c_to_ri1 : casper_library/Misc/c_to_ri  SystemSampleTime=-1  n_bits=BitWidth  bin_pt=BitWidth-1
      settings: AttributesFormatString=8_7 r/i
  ri_to_c : casper_library/Misc/ri_to_c  SystemSampleTime=-1
  a+b : Outport  OutDataType=sfix(16)  OutScaling=2^0
  wires:
  Scale/1 -> Convert2/1
  Scale1/1 -> Convert/1
  b/1 -> c_to_ri1/1
  ri_to_c/1 -> a+b/1
  a/1 -> c_to_ri/1
  Convert2/1 -> ri_to_c/2
  Convert/1 -> ri_to_c/1
  c_to_ri1/2 -> AddSub2/2
  c_to_ri1/1 -> AddSub/2
  c_to_ri/2 -> AddSub2/1
  c_to_ri/1 -> AddSub/1
  AddSub2/1 -> Scale/1
  AddSub/1 -> Scale1/1

== system ox_lib/8pt_fft/cplx_add7 ==
  a : Inport  OutDataType=sfix(16)  OutScaling=2^0
  b : Inport  Port=2  OutDataType=sfix(16)  OutScaling=2^0
  AddSub : xbsIndex_r4/AddSub  mode=Addition  use_carryin=off  use_carryout=off  en=off  latency=add_latency  precision=Full  arith_type=Unsigned  n_bits=8  bin_pt=2  quantization=Truncate  overflow=Wrap  dbl_ovrd=off  use_behavioral_HDL=on  hw_selection=Fabric  pipelined=off  use_rpm=on  block_type=addsub
      settings: xl_area=[0, 0, 0, 0, 0, 0, 0]  block_version=9.1.01
  AddSub2 : xbsIndex_r4/AddSub  mode=Addition  use_carryin=off  use_carryout=off  en=off  latency=add_latency  precision=Full  arith_type=Unsigned  n_bits=8  bin_pt=2  quantization=Truncate  overflow=Wrap  dbl_ovrd=off  use_behavioral_HDL=on  hw_selection=Fabric  pipelined=off  use_rpm=on  block_type=addsub
      settings: xl_area=[0, 0, 0, 0, 0, 0, 0]  block_version=9.1.01
  Convert : xbsIndex_r4/Convert  arith_type="Signed  (2's comp)"  n_bits=BitWidth  bin_pt=BitWidth - 1  quantization="Round  (unbiased: +/- Inf)"  overflow=Saturate  latency=add_latency  dbl_ovrd=off  pipeline=off  block_type=convert
      settings: xl_area=[0, 0, 0, 0, 0, 0, 0]
  Convert2 : xbsIndex_r4/Convert  arith_type="Signed  (2's comp)"  n_bits=BitWidth  bin_pt=BitWidth - 1  quantization="Round  (unbiased: +/- Inf)"  overflow=Saturate  latency=add_latency  dbl_ovrd=off  pipeline=off  block_type=convert
      settings: xl_area=[0, 0, 0, 0, 0, 0, 0]
  Scale : xbsIndex_r4/Scale  scale_factor=-1  dbl_ovrd=off  block_type=scale
  Scale1 : xbsIndex_r4/Scale  scale_factor=-1  dbl_ovrd=off  block_type=scale
  c_to_ri : casper_library/Misc/c_to_ri  SystemSampleTime=-1  n_bits=BitWidth  bin_pt=BitWidth-1
      settings: AttributesFormatString=8_7 r/i
  c_to_ri1 : casper_library/Misc/c_to_ri  SystemSampleTime=-1  n_bits=BitWidth  bin_pt=BitWidth-1
      settings: AttributesFormatString=8_7 r/i
  ri_to_c : casper_library/Misc/ri_to_c  SystemSampleTime=-1
  a+b : Outport  OutDataType=sfix(16)  OutScaling=2^0
  wires:
  AddSub/1 -> Scale1/1
  AddSub2/1 -> Scale/1
  c_to_ri/1 -> AddSub/1
  c_to_ri/2 -> AddSub2/1
  c_to_ri1/1 -> AddSub/2
  c_to_ri1/2 -> AddSub2/2
  Convert/1 -> ri_to_c/1
  Convert2/1 -> ri_to_c/2
  a/1 -> c_to_ri/1
  ri_to_c/1 -> a+b/1
  b/1 -> c_to_ri1/1
  Scale1/1 -> Convert/1
  Scale/1 -> Convert2/1

== system ox_lib/8pt_fft/cplx_add8 ==
  a : Inport  OutDataType=sfix(16)  OutScaling=2^0
  b : Inport  Port=2  OutDataType=sfix(16)  OutScaling=2^0
  AddSub : xbsIndex_r4/AddSub  mode=Addition  use_carryin=off  use_carryout=off  en=off  latency=add_latency  precision=Full  arith_type=Unsigned  n_bits=8  bin_pt=2  quantization=Truncate  overflow=Wrap  dbl_ovrd=off  use_behavioral_HDL=on  hw_selection=Fabric  pipelined=off  use_rpm=on  block_type=addsub
      settings: xl_area=[0, 0, 0, 0, 0, 0, 0]  block_version=9.1.01
  AddSub2 : xbsIndex_r4/AddSub  mode=Addition  use_carryin=off  use_carryout=off  en=off  latency=add_latency  precision=Full  arith_type=Unsigned  n_bits=8  bin_pt=2  quantization=Truncate  overflow=Wrap  dbl_ovrd=off  use_behavioral_HDL=on  hw_selection=Fabric  pipelined=off  use_rpm=on  block_type=addsub
      settings: xl_area=[0, 0, 0, 0, 0, 0, 0]  block_version=9.1.01
  Convert : xbsIndex_r4/Convert  arith_type="Signed  (2's comp)"  n_bits=BitWidth  bin_pt=BitWidth - 1  quantization="Round  (unbiased: +/- Inf)"  overflow=Saturate  latency=add_latency  dbl_ovrd=off  pipeline=off  block_type=convert
      settings: xl_area=[0, 0, 0, 0, 0, 0, 0]
  Convert2 : xbsIndex_r4/Convert  arith_type="Signed  (2's comp)"  n_bits=BitWidth  bin_pt=BitWidth - 1  quantization="Round  (unbiased: +/- Inf)"  overflow=Saturate  latency=add_latency  dbl_ovrd=off  pipeline=off  block_type=convert
      settings: xl_area=[0, 0, 0, 0, 0, 0, 0]
  Scale : xbsIndex_r4/Scale  scale_factor=-1  dbl_ovrd=off  block_type=scale
  Scale1 : xbsIndex_r4/Scale  scale_factor=-1  dbl_ovrd=off  block_type=scale
  c_to_ri : casper_library/Misc/c_to_ri  SystemSampleTime=-1  n_bits=BitWidth  bin_pt=BitWidth-1
      settings: AttributesFormatString=8_7 r/i
  c_to_ri1 : casper_library/Misc/c_to_ri  SystemSampleTime=-1  n_bits=BitWidth  bin_pt=BitWidth-1
      settings: AttributesFormatString=8_7 r/i
  ri_to_c : casper_library/Misc/ri_to_c  SystemSampleTime=-1
  a+b : Outport  OutDataType=sfix(16)  OutScaling=2^0
  wires:
  Scale/1 -> Convert2/1
  Scale1/1 -> Convert/1
  b/1 -> c_to_ri1/1
  ri_to_c/1 -> a+b/1
  a/1 -> c_to_ri/1
  Convert2/1 -> ri_to_c/2
  Convert/1 -> ri_to_c/1
  c_to_ri1/2 -> AddSub2/2
  c_to_ri1/1 -> AddSub/2
  c_to_ri/2 -> AddSub2/1
  c_to_ri/1 -> AddSub/1
  AddSub2/1 -> Scale/1
  AddSub/1 -> Scale1/1

== system ox_lib/8pt_fft/twid1 ==
  In1 : Inport  OutDataType=sfix(16)  OutScaling=2^0
  cmult : Subsystem  AncestorBlock=casper_library/Multipliers/cmult  mask(Complex Multiplier (4 real multipliers)){n_bits_a=8, bin_pt_a=7, n_bits_b=8, bin_pt_b=7, n_bits_ab=8, bin_pt_ab=7, quantization=Round  (unbiased: +/- Inf), overflow=Saturate, mult_latency=3, add_latency=2}
      mask prompts: n_bits_a "Number of Bits 'a'"; bin_pt_a "Binary Point 'a'"; n_bits_b "Number of Bits 'b'"; bin_pt_b "Binary Point 'b'"; n_bits_ab "Number of Bits 'ab'"; bin_pt_ab "Binary Point 'ab'"; mult_latency "Multiplier Latency"; add_latency "Adder Latency"
      mask help:
      | This block multiplies two complex numbers using 4 real multipliers and 2 real adders.
      |
      | Latency = multiplier latency + adder latency.
      mask init:
      | cmult_init(gcb, ...
      |     'n_bits_a',n_bits_a, ...
      |     'bin_pt_a',bin_pt_a, ...
      |     'n_bits_b',n_bits_b, ...
      |     'bin_pt_b',bin_pt_b, ...
      |     'n_bits_ab',n_bits_ab, ...
      |     'bin_pt_ab',bin_pt_ab, ...
      |     'quantization',quantization, ...
      |     'overflow', overflow,...
      |     'mult_latency', mult_latency, ...
      |     'add_latency', add_latency);
      settings: AttributesFormatString=|
      | 8_7 * 8_7 ==> 8_7
      | round inf, saturate
      |  Latency: 8
      mask StyleString: edit,edit,edit,edit,edit,edit,popup(Truncate|Round  (unbiased: +/- Inf)|Round  (unbiased: Even Values)),popup(Wrap|Saturate|Error),edit,edit
  im : xbsIndex_r4/Constant  arith_type=Signed (2's comp)  const=sin(phase)  n_bits=8  bin_pt=7  explicit_period=on  period=1  equ=P=C  opselect=C  inp2=PCIN>>17  opr=+  inp1=P  carry=CIN  dbl_ovrd=off  block_type=constant
      settings: block_version=11.4
  re : xbsIndex_r4/Constant  arith_type=Signed (2's comp)  const=cos(phase)  n_bits=8  bin_pt=7  explicit_period=on  period=1  equ=P=C  opselect=C  inp2=PCIN>>17  opr=+  inp1=P  carry=CIN  dbl_ovrd=off  block_type=constant
      settings: block_version=11.4
  ri_to_c1 : casper_library/Misc/ri_to_c  SystemSampleTime=-1
  Out1 : Outport  OutDataType=sfix(16)  OutScaling=2^0
  wires:
  cmult/1(ab) -> Out1/1
  In1/1 -> cmult/1(a)
  ri_to_c1/1 -> cmult/2(b)
  im/1 -> ri_to_c1/2
  re/1 -> ri_to_c1/1

== system ox_lib/8pt_fft/twid2 ==
  In1 : Inport  OutDataType=sfix(16)  OutScaling=2^0
  cmult : Subsystem  AncestorBlock=casper_library/Multipliers/cmult  mask(Complex Multiplier (4 real multipliers)){n_bits_a=8, bin_pt_a=7, n_bits_b=8, bin_pt_b=7, n_bits_ab=8, bin_pt_ab=7, quantization=Round  (unbiased: +/- Inf), overflow=Saturate, mult_latency=3, add_latency=2}
      mask prompts: n_bits_a "Number of Bits 'a'"; bin_pt_a "Binary Point 'a'"; n_bits_b "Number of Bits 'b'"; bin_pt_b "Binary Point 'b'"; n_bits_ab "Number of Bits 'ab'"; bin_pt_ab "Binary Point 'ab'"; mult_latency "Multiplier Latency"; add_latency "Adder Latency"
      mask help:
      | This block multiplies two complex numbers using 4 real multipliers and 2 real adders.
      |
      | Latency = multiplier latency + adder latency.
      mask init: same as ox_lib/8pt_fft/twid1/cmult
      settings: AttributesFormatString=|
      | 8_7 * 8_7 ==> 8_7
      | round inf, saturate
      |  Latency: 8
      mask StyleString: edit,edit,edit,edit,edit,edit,popup(Truncate|Round  (unbiased: +/- Inf)|Round  (unbiased: Even Values)),popup(Wrap|Saturate|Error),edit,edit
  im : xbsIndex_r4/Constant  arith_type=Signed (2's comp)  const=sin(phase)  n_bits=8  bin_pt=7  explicit_period=on  period=1  equ=P=C  opselect=C  inp2=PCIN>>17  opr=+  inp1=P  carry=CIN  dbl_ovrd=off  block_type=constant
      settings: block_version=11.4
  re : xbsIndex_r4/Constant  arith_type=Signed (2's comp)  const=cos(phase)  n_bits=8  bin_pt=7  explicit_period=on  period=1  equ=P=C  opselect=C  inp2=PCIN>>17  opr=+  inp1=P  carry=CIN  dbl_ovrd=off  block_type=constant
      settings: block_version=11.4
  ri_to_c1 : casper_library/Misc/ri_to_c  SystemSampleTime=-1
  Out1 : Outport  OutDataType=sfix(16)  OutScaling=2^0
  wires:
  re/1 -> ri_to_c1/1
  im/1 -> ri_to_c1/2
  ri_to_c1/1 -> cmult/2(b)
  In1/1 -> cmult/1(a)
  cmult/1(ab) -> Out1/1

== system ox_lib/8pt_fft/twid3 ==
  In1 : Inport  OutDataType=sfix(16)  OutScaling=2^0
  cmult : Subsystem  AncestorBlock=casper_library/Multipliers/cmult  mask(Complex Multiplier (4 real multipliers)){n_bits_a=8, bin_pt_a=7, n_bits_b=8, bin_pt_b=7, n_bits_ab=8, bin_pt_ab=7, quantization=Round  (unbiased: +/- Inf), overflow=Saturate, mult_latency=3, add_latency=2}
      mask prompts: n_bits_a "Number of Bits 'a'"; bin_pt_a "Binary Point 'a'"; n_bits_b "Number of Bits 'b'"; bin_pt_b "Binary Point 'b'"; n_bits_ab "Number of Bits 'ab'"; bin_pt_ab "Binary Point 'ab'"; mult_latency "Multiplier Latency"; add_latency "Adder Latency"
      mask help:
      | This block multiplies two complex numbers using 4 real multipliers and 2 real adders.
      |
      | Latency = multiplier latency + adder latency.
      mask init: same as ox_lib/8pt_fft/twid1/cmult
      settings: AttributesFormatString=|
      | 8_7 * 8_7 ==> 8_7
      | round inf, saturate
      |  Latency: 8
      mask StyleString: edit,edit,edit,edit,edit,edit,popup(Truncate|Round  (unbiased: +/- Inf)|Round  (unbiased: Even Values)),popup(Wrap|Saturate|Error),edit,edit
  im : xbsIndex_r4/Constant  arith_type=Signed (2's comp)  const=sin(phase)  n_bits=8  bin_pt=7  explicit_period=on  period=1  equ=P=C  opselect=C  inp2=PCIN>>17  opr=+  inp1=P  carry=CIN  dbl_ovrd=off  block_type=constant
      settings: block_version=11.4
  re : xbsIndex_r4/Constant  arith_type=Signed (2's comp)  const=cos(phase)  n_bits=8  bin_pt=7  explicit_period=on  period=1  equ=P=C  opselect=C  inp2=PCIN>>17  opr=+  inp1=P  carry=CIN  dbl_ovrd=off  block_type=constant
      settings: block_version=11.4
  ri_to_c1 : casper_library/Misc/ri_to_c  SystemSampleTime=-1
  Out1 : Outport  OutDataType=sfix(16)  OutScaling=2^0
  wires:
  cmult/1(ab) -> Out1/1
  In1/1 -> cmult/1(a)
  ri_to_c1/1 -> cmult/2(b)
  im/1 -> ri_to_c1/2
  re/1 -> ri_to_c1/1

== system ox_lib/8pt_fft/twid4 ==
  In1 : Inport  OutDataType=sfix(16)  OutScaling=2^0
  cmult : Subsystem  AncestorBlock=casper_library/Multipliers/cmult  mask(Complex Multiplier (4 real multipliers)){n_bits_a=8, bin_pt_a=7, n_bits_b=8, bin_pt_b=7, n_bits_ab=8, bin_pt_ab=7, quantization=Round  (unbiased: +/- Inf), overflow=Saturate, mult_latency=3, add_latency=2}
      mask prompts: n_bits_a "Number of Bits 'a'"; bin_pt_a "Binary Point 'a'"; n_bits_b "Number of Bits 'b'"; bin_pt_b "Binary Point 'b'"; n_bits_ab "Number of Bits 'ab'"; bin_pt_ab "Binary Point 'ab'"; mult_latency "Multiplier Latency"; add_latency "Adder Latency"
      mask help:
      | This block multiplies two complex numbers using 4 real multipliers and 2 real adders.
      |
      | Latency = multiplier latency + adder latency.
      mask init: same as ox_lib/8pt_fft/twid1/cmult
      settings: AttributesFormatString=|
      | 8_7 * 8_7 ==> 8_7
      | round inf, saturate
      |  Latency: 8
      mask StyleString: edit,edit,edit,edit,edit,edit,popup(Truncate|Round  (unbiased: +/- Inf)|Round  (unbiased: Even Values)),popup(Wrap|Saturate|Error),edit,edit
  im : xbsIndex_r4/Constant  arith_type=Signed (2's comp)  const=sin(phase)  n_bits=8  bin_pt=7  explicit_period=on  period=1  equ=P=C  opselect=C  inp2=PCIN>>17  opr=+  inp1=P  carry=CIN  dbl_ovrd=off  block_type=constant
      settings: block_version=11.4
  re : xbsIndex_r4/Constant  arith_type=Signed (2's comp)  const=cos(phase)  n_bits=8  bin_pt=7  explicit_period=on  period=1  equ=P=C  opselect=C  inp2=PCIN>>17  opr=+  inp1=P  carry=CIN  dbl_ovrd=off  block_type=constant
      settings: block_version=11.4
  ri_to_c1 : casper_library/Misc/ri_to_c  SystemSampleTime=-1
  Out1 : Outport  OutDataType=sfix(16)  OutScaling=2^0
  wires:
  re/1 -> ri_to_c1/1
  im/1 -> ri_to_c1/2
  ri_to_c1/1 -> cmult/2(b)
  In1/1 -> cmult/1(a)
  cmult/1(ab) -> Out1/1

== system ox_lib/8pt_fft/twid5 ==
  In1 : Inport  OutDataType=sfix(16)  OutScaling=2^0
  cmult : Subsystem  AncestorBlock=casper_library/Multipliers/cmult  mask(Complex Multiplier (4 real multipliers)){n_bits_a=8, bin_pt_a=7, n_bits_b=8, bin_pt_b=7, n_bits_ab=8, bin_pt_ab=7, quantization=Round  (unbiased: +/- Inf), overflow=Saturate, mult_latency=3, add_latency=2}
      mask prompts: n_bits_a "Number of Bits 'a'"; bin_pt_a "Binary Point 'a'"; n_bits_b "Number of Bits 'b'"; bin_pt_b "Binary Point 'b'"; n_bits_ab "Number of Bits 'ab'"; bin_pt_ab "Binary Point 'ab'"; mult_latency "Multiplier Latency"; add_latency "Adder Latency"
      mask help:
      | This block multiplies two complex numbers using 4 real multipliers and 2 real adders.
      |
      | Latency = multiplier latency + adder latency.
      mask init: same as ox_lib/8pt_fft/twid1/cmult
      settings: AttributesFormatString=|
      | 8_7 * 8_7 ==> 8_7
      | round inf, saturate
      |  Latency: 8
      mask StyleString: edit,edit,edit,edit,edit,edit,popup(Truncate|Round  (unbiased: +/- Inf)|Round  (unbiased: Even Values)),popup(Wrap|Saturate|Error),edit,edit
  im : xbsIndex_r4/Constant  arith_type=Signed (2's comp)  const=sin(phase)  n_bits=8  bin_pt=7  explicit_period=on  period=1  equ=P=C  opselect=C  inp2=PCIN>>17  opr=+  inp1=P  carry=CIN  dbl_ovrd=off  block_type=constant
      settings: block_version=11.4
  re : xbsIndex_r4/Constant  arith_type=Signed (2's comp)  const=cos(phase)  n_bits=8  bin_pt=7  explicit_period=on  period=1  equ=P=C  opselect=C  inp2=PCIN>>17  opr=+  inp1=P  carry=CIN  dbl_ovrd=off  block_type=constant
      settings: block_version=11.4
  ri_to_c1 : casper_library/Misc/ri_to_c  SystemSampleTime=-1
  Out1 : Outport  OutDataType=sfix(16)  OutScaling=2^0
  wires:
  cmult/1(ab) -> Out1/1
  In1/1 -> cmult/1(a)
  ri_to_c1/1 -> cmult/2(b)
  im/1 -> ri_to_c1/2
  re/1 -> ri_to_c1/1

== system ox_lib/8pt_fft/twid6 ==
  In1 : Inport  OutDataType=sfix(16)  OutScaling=2^0
  cmult : Subsystem  AncestorBlock=casper_library/Multipliers/cmult  mask(Complex Multiplier (4 real multipliers)){n_bits_a=8, bin_pt_a=7, n_bits_b=8, bin_pt_b=7, n_bits_ab=8, bin_pt_ab=7, quantization=Round  (unbiased: +/- Inf), overflow=Saturate, mult_latency=3, add_latency=2}
      mask prompts: n_bits_a "Number of Bits 'a'"; bin_pt_a "Binary Point 'a'"; n_bits_b "Number of Bits 'b'"; bin_pt_b "Binary Point 'b'"; n_bits_ab "Number of Bits 'ab'"; bin_pt_ab "Binary Point 'ab'"; mult_latency "Multiplier Latency"; add_latency "Adder Latency"
      mask help:
      | This block multiplies two complex numbers using 4 real multipliers and 2 real adders.
      |
      | Latency = multiplier latency + adder latency.
      mask init: same as ox_lib/8pt_fft/twid1/cmult
      settings: AttributesFormatString=|
      | 8_7 * 8_7 ==> 8_7
      | round inf, saturate
      |  Latency: 8
      mask StyleString: edit,edit,edit,edit,edit,edit,popup(Truncate|Round  (unbiased: +/- Inf)|Round  (unbiased: Even Values)),popup(Wrap|Saturate|Error),edit,edit
  im : xbsIndex_r4/Constant  arith_type=Signed (2's comp)  const=sin(phase)  n_bits=8  bin_pt=7  explicit_period=on  period=1  equ=P=C  opselect=C  inp2=PCIN>>17  opr=+  inp1=P  carry=CIN  dbl_ovrd=off  block_type=constant
      settings: block_version=11.4
  re : xbsIndex_r4/Constant  arith_type=Signed (2's comp)  const=cos(phase)  n_bits=8  bin_pt=7  explicit_period=on  period=1  equ=P=C  opselect=C  inp2=PCIN>>17  opr=+  inp1=P  carry=CIN  dbl_ovrd=off  block_type=constant
      settings: block_version=11.4
  ri_to_c1 : casper_library/Misc/ri_to_c  SystemSampleTime=-1
  Out1 : Outport  OutDataType=sfix(16)  OutScaling=2^0
  wires:
  re/1 -> ri_to_c1/1
  im/1 -> ri_to_c1/2
  ri_to_c1/1 -> cmult/2(b)
  In1/1 -> cmult/1(a)
  cmult/1(ab) -> Out1/1

== system ox_lib/8pt_fft/twid8 ==
  In1 : Inport  OutDataType=sfix(16)  OutScaling=2^0
  cmult : Subsystem  AncestorBlock=casper_library/Multipliers/cmult  mask(Complex Multiplier (4 real multipliers)){n_bits_a=8, bin_pt_a=7, n_bits_b=8, bin_pt_b=7, n_bits_ab=8, bin_pt_ab=7, quantization=Round  (unbiased: +/- Inf), overflow=Saturate, mult_latency=3, add_latency=2}
      mask prompts: n_bits_a "Number of Bits 'a'"; bin_pt_a "Binary Point 'a'"; n_bits_b "Number of Bits 'b'"; bin_pt_b "Binary Point 'b'"; n_bits_ab "Number of Bits 'ab'"; bin_pt_ab "Binary Point 'ab'"; mult_latency "Multiplier Latency"; add_latency "Adder Latency"
      mask help:
      | This block multiplies two complex numbers using 4 real multipliers and 2 real adders.
      |
      | Latency = multiplier latency + adder latency.
      mask init: same as ox_lib/8pt_fft/twid1/cmult
      settings: AttributesFormatString=|
      | 8_7 * 8_7 ==> 8_7
      | round inf, saturate
      |  Latency: 8
      mask StyleString: edit,edit,edit,edit,edit,edit,popup(Truncate|Round  (unbiased: +/- Inf)|Round  (unbiased: Even Values)),popup(Wrap|Saturate|Error),edit,edit
  im : xbsIndex_r4/Constant  arith_type=Signed (2's comp)  const=sin(phase)  n_bits=8  bin_pt=7  explicit_period=on  period=1  equ=P=C  opselect=C  inp2=PCIN>>17  opr=+  inp1=P  carry=CIN  dbl_ovrd=off  block_type=constant
      settings: block_version=11.4
  re : xbsIndex_r4/Constant  arith_type=Signed (2's comp)  const=cos(phase)  n_bits=8  bin_pt=7  explicit_period=on  period=1  equ=P=C  opselect=C  inp2=PCIN>>17  opr=+  inp1=P  carry=CIN  dbl_ovrd=off  block_type=constant
      settings: block_version=11.4
  ri_to_c1 : casper_library/Misc/ri_to_c  SystemSampleTime=-1
  Out1 : Outport  OutDataType=sfix(16)  OutScaling=2^0
  wires:
  re/1 -> ri_to_c1/1
  im/1 -> ri_to_c1/2
  ri_to_c1/1 -> cmult/2(b)
  In1/1 -> cmult/1(a)
  cmult/1(ab) -> Out1/1
